simulink model "filtros4"  (R2018b)
settings: Solver=VariableStepAuto  StartTime=0.0  StopTime=10.0  RelTol=1e-3
(part 3 of 3)

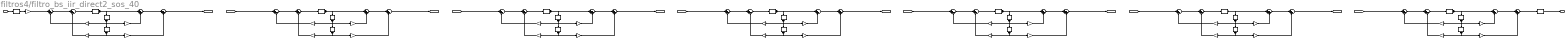
== system filtros4/filtro_bs_iir_direct2_sos_40 ==
  Input : Inport
  CastState{1..7} (7 alike) : DataTypeConversion  OutDataTypeStr=fixdt(1,16,15)  RndMeth=Convergent
  ConvertIn : DataTypeConversion  OutDataTypeStr=fixdt(1,16,15)  RndMeth=Nearest  SaturateOnIntegerOverflow=on
  ConvertOut : DataTypeConversion  OutDataTypeStr=fixdt(1,16,11)  RndMeth=Convergent
  Delay{11..17,21..27} (14 alike) : Delay  DelayLength=1  InitialCondition=0
  SumA{21..27,31..37} (14 alike) : Sum  Inputs=|+-  AccumDataTypeStr=fixdt(1,40,35)  OutDataTypeStr=fixdt(1,40,35)  RndMeth=Convergent
  SumB{21..27,31..37} (14 alike) : Sum  Inputs=|++  AccumDataTypeStr=fixdt(1,40,35)  OutDataTypeStr=fixdt(1,40,35)  RndMeth=Convergent
  a(2)(1) : Gain  Gain=-0.813428281179642165  ParamDataTypeStr=fixdt(1,40,38)  OutDataTypeStr=fixdt(1,56,53)  RndMeth=Convergent
  a(2)(2) : Gain  Gain=-0.742197661664668717  ParamDataTypeStr=fixdt(1,40,38)  OutDataTypeStr=fixdt(1,56,53)  RndMeth=Convergent
  a(2)(3) : Gain  Gain=-1.18020037227255226  ParamDataTypeStr=fixdt(1,40,38)  OutDataTypeStr=fixdt(1,56,53)  RndMeth=Convergent
  a(2)(4) : Gain  Gain=-0.8635074436780521  ParamDataTypeStr=fixdt(1,40,38)  OutDataTypeStr=fixdt(1,56,53)  RndMeth=Convergent
  a(2)(5) : Gain  Gain=-1.17581613832315401  ParamDataTypeStr=fixdt(1,40,38)  OutDataTypeStr=fixdt(1,56,53)  RndMeth=Convergent
  a(2)(6) : Gain  Gain=-0.90563072038096426  ParamDataTypeStr=fixdt(1,40,38)  OutDataTypeStr=fixdt(1,56,53)  RndMeth=Convergent
  a(2)(7) : Gain  Gain=-1.16875024700793517  ParamDataTypeStr=fixdt(1,40,38)  OutDataTypeStr=fixdt(1,56,53)  RndMeth=Convergent
  a(3)(1) : Gain  Gain=0.552005579906472033  ParamDataTypeStr=fixdt(1,40,38)  OutDataTypeStr=fixdt(1,56,53)  RndMeth=Convergent
  a(3)(2) : Gain  Gain=0.854865767395351028  ParamDataTypeStr=fixdt(1,40,38)  OutDataTypeStr=fixdt(1,56,53)  RndMeth=Convergent
  a(3)(3) : Gain  Gain=0.875550994084790757  ParamDataTypeStr=fixdt(1,40,38)  OutDataTypeStr=fixdt(1,56,53)  RndMeth=Convergent
  a(3)(4) : Gain  Gain=0.959930995951585597  ParamDataTypeStr=fixdt(1,40,38)  OutDataTypeStr=fixdt(1,56,53)  RndMeth=Convergent
  a(3)(5) : Gain  Gain=0.964163580544992183  ParamDataTypeStr=fixdt(1,40,38)  OutDataTypeStr=fixdt(1,56,53)  RndMeth=Convergent
  a(3)(6) : Gain  Gain=0.990340187952881257  ParamDataTypeStr=fixdt(1,40,38)  OutDataTypeStr=fixdt(1,56,53)  RndMeth=Convergent
  a(3)(7) : Gain  Gain=0.991207917022611129  ParamDataTypeStr=fixdt(1,40,38)  OutDataTypeStr=fixdt(1,56,53)  RndMeth=Convergent
  b(2)(1) : Gain  Gain=-1.11152954346655419  ParamDataTypeStr=fixdt(1,40,38)  OutDataTypeStr=fixdt(1,56,53)  RndMeth=Convergent
  b(2)(2) : Gain  Gain=-1.07211536629555804  ParamDataTypeStr=fixdt(1,40,38)  OutDataTypeStr=fixdt(1,56,53)  RndMeth=Convergent
  b(2)(3) : Gain  Gain=-1.0032399136855954  ParamDataTypeStr=fixdt(1,40,38)  OutDataTypeStr=fixdt(1,56,53)  RndMeth=Convergent
  b(2)(4) : Gain  Gain=-1.01063368621325411  ParamDataTypeStr=fixdt(1,40,38)  OutDataTypeStr=fixdt(1,56,53)  RndMeth=Convergent
  b(2)(5) : Gain  Gain=-1.05770999558857559  ParamDataTypeStr=fixdt(1,40,38)  OutDataTypeStr=fixdt(1,56,53)  RndMeth=Convergent
  b(2)(6) : Gain  Gain=-0.980405596804986956  ParamDataTypeStr=fixdt(1,40,38)  OutDataTypeStr=fixdt(1,56,53)  RndMeth=Convergent
  b(2)(7) : Gain  Gain=-1.1019651730511173  ParamDataTypeStr=fixdt(1,40,38)  OutDataTypeStr=fixdt(1,56,53)  RndMeth=Convergent
  b(3)(1) : Gain  Gain=1.05088219447620013  ParamDataTypeStr=fixdt(1,40,38)  OutDataTypeStr=fixdt(1,56,53)  RndMeth=Convergent
  b(3)(2) : Gain  Gain=1.06865251897541036  ParamDataTypeStr=fixdt(1,40,38)  OutDataTypeStr=fixdt(1,56,53)  RndMeth=Convergent
  b(3)(3) : Gain  Gain=0.935758131903575485  ParamDataTypeStr=fixdt(1,40,38)  OutDataTypeStr=fixdt(1,56,53)  RndMeth=Convergent
  b(3)(4) : Gain  Gain=1.03083232416279569  ParamDataTypeStr=fixdt(1,40,38)  OutDataTypeStr=fixdt(1,56,53)  RndMeth=Convergent
  b(3)(5) : Gain  Gain=0.951581007807177359  ParamDataTypeStr=fixdt(1,40,38)  OutDataTypeStr=fixdt(1,56,53)  RndMeth=Convergent
  b(3)(6) : Gain  Gain=0.97009053687980229  ParamDataTypeStr=fixdt(1,40,38)  OutDataTypeStr=fixdt(1,56,53)  RndMeth=Convergent
  b(3)(7) : Gain  Gain=0.999999494703609493  ParamDataTypeStr=fixdt(1,40,38)  OutDataTypeStr=fixdt(1,56,53)  RndMeth=Convergent
  s(1) : Gain  Gain=0.619240669533610344  ParamDataTypeStr=fixdt(1,40,39)  OutDataTypeStr=fixdt(1,16,10)  RndMeth=Convergent
  Output : Outport
  wires:
  Input/1 -> ConvertIn/1
  s(1)/1 -> SumA21/1
  SumA21/1 -> SumA31/1
  SumA31/1 -> CastState1/1
  CastState1/1 -> SumB21/1, Delay11/1
  SumB21/1 -> SumB31/1
  SumB31/1 -> [Sect1]
  a(2)(1)/1 -> SumA21/2
  Delay11/1 -> a(2)(1)/1, b(2)(1)/1, Delay21/1
  b(2)(1)/1 -> SumB21/2
  a(3)(1)/1 -> SumA31/2
  Delay21/1 -> a(3)(1)/1, b(3)(1)/1
  b(3)(1)/1 -> SumB31/2
  ConvertIn/1 -> s(1)/1
  [Sect1] -> SumA22/1
  SumA22/1 -> SumA32/1
  SumA32/1 -> CastState2/1
  CastState2/1 -> SumB22/1, Delay12/1
  SumB22/1 -> SumB32/1
  SumB32/1 -> [Sect2]
  a(2)(2)/1 -> SumA22/2
  Delay12/1 -> a(2)(2)/1, b(2)(2)/1, Delay22/1
  b(2)(2)/1 -> SumB22/2
  a(3)(2)/1 -> SumA32/2
  Delay22/1 -> a(3)(2)/1, b(3)(2)/1
  b(3)(2)/1 -> SumB32/2
  [Sect2] -> SumA23/1
  SumA23/1 -> SumA33/1
  SumA33/1 -> CastState3/1
  CastState3/1 -> SumB23/1, Delay13/1
  SumB23/1 -> SumB33/1
  SumB33/1 -> [Sect3]
  a(2)(3)/1 -> SumA23/2
  Delay13/1 -> a(2)(3)/1, b(2)(3)/1, Delay23/1
  b(2)(3)/1 -> SumB23/2
  a(3)(3)/1 -> SumA33/2
  Delay23/1 -> a(3)(3)/1, b(3)(3)/1
  b(3)(3)/1 -> SumB33/2
  [Sect3] -> SumA24/1
  SumA24/1 -> SumA34/1
  SumA34/1 -> CastState4/1
  CastState4/1 -> SumB24/1, Delay14/1
  SumB24/1 -> SumB34/1
  SumB34/1 -> [Sect4]
  a(2)(4)/1 -> SumA24/2
  Delay14/1 -> a(2)(4)/1, b(2)(4)/1, Delay24/1
  b(2)(4)/1 -> SumB24/2
  a(3)(4)/1 -> SumA34/2
  Delay24/1 -> a(3)(4)/1, b(3)(4)/1
  b(3)(4)/1 -> SumB34/2
  [Sect4] -> SumA25/1
  SumA25/1 -> SumA35/1
  SumA35/1 -> CastState5/1
  CastState5/1 -> SumB25/1, Delay15/1
  SumB25/1 -> SumB35/1
  SumB35/1 -> [Sect5]
  a(2)(5)/1 -> SumA25/2
  Delay15/1 -> a(2)(5)/1, b(2)(5)/1, Delay25/1
  b(2)(5)/1 -> SumB25/2
  a(3)(5)/1 -> SumA35/2
  Delay25/1 -> a(3)(5)/1, b(3)(5)/1
  b(3)(5)/1 -> SumB35/2
  [Sect5] -> SumA26/1
  SumA26/1 -> SumA36/1
  SumA36/1 -> CastState6/1
  CastState6/1 -> SumB26/1, Delay16/1
  SumB26/1 -> SumB36/1
  SumB36/1 -> [Sect6]
  a(2)(6)/1 -> SumA26/2
  Delay16/1 -> a(2)(6)/1, b(2)(6)/1, Delay26/1
  b(2)(6)/1 -> SumB26/2
  a(3)(6)/1 -> SumA36/2
  Delay26/1 -> a(3)(6)/1, b(3)(6)/1
  b(3)(6)/1 -> SumB36/2
  [Sect6] -> SumA27/1
  SumA27/1 -> SumA37/1
  SumA37/1 -> CastState7/1
  CastState7/1 -> SumB27/1, Delay17/1
  SumB27/1 -> SumB37/1
  SumB37/1 -> ConvertOut/1
  a(2)(7)/1 -> SumA27/2
  Delay17/1 -> a(2)(7)/1, b(2)(7)/1, Delay27/1
  b(2)(7)/1 -> SumB27/2
  a(3)(7)/1 -> SumA37/2
  Delay27/1 -> a(3)(7)/1, b(3)(7)/1
  b(3)(7)/1 -> SumB37/2
  ConvertOut/1 -> Output/1
